simulink model "SensorModelSim"  (R2019b)
settings: Solver=VariableStepAuto  StartTime=0.0  StopTime=10.0  RelTol=1e-3
values from neighbouring files (symbols this model uses):
  A = [0  0  0  1  0  0  0  0  0  0  0  0 ... (first row only)    [LQR.m]    (also in LQR_Goal_1.m; Naman_LQR_Working.m; PlantModel.m = [0  0  0  1  0  0  0  0  0  0  0  0;      0  0  0  0  1  0  )
  B = [0      0       0       0 ... (first row only)    [LQR.m]    (also in LQR_Goal_1.m; Naman_LQR_Working.m; PlantModel.m = [0 0 0 0;      0 0 0 0;      0 0 0 0;      0 0 0 0;      0 0)
  C = [1 0 0 0 0 0 0 0 0 0 0 0 ... (first row only)    [LQR.m]    (also in LQR_Goal_1.m; Naman_LQR_Working.m; PlantModel.m = [1 0 0 0 0 0 0 0 0 0 0 0;      0 1 0 0 0 0 0 0 0 0 0 0;     )
  D = zeros(6,4)    [LQR.m]    (also in LQR_Goal_1.m; Naman_LQR_Working.m; PlantModel.m)
settings Model: Creator=Lakshu  LastModifiedBy=Sravan

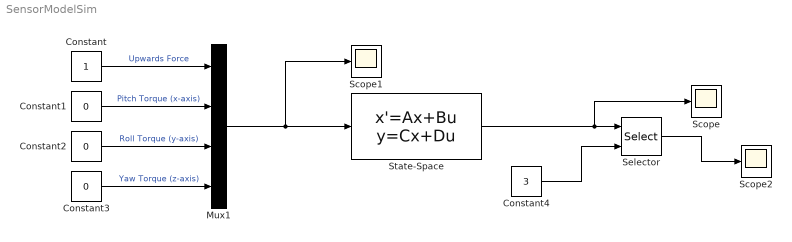
== system SensorModelSim ==
  Constant : Constant
  Constant1 : Constant  Value=0
  Constant2 : Constant  Value=0
  Constant3 : Constant  Value=0
  Constant4 : Constant  Value=3
  Mux1 : Mux
  Scope : Scope
  Scope1 : Scope
  Scope2 : Scope
  Selector : Selector  InputPortWidth=6  IndexOptions=Index vector (port)  Indices=[2]  OutputSizes=1
  State-Space : StateSpace  A=A  B=B  C=C  D=D  InitialCondition=0
  wires:
  Mux1/1 -> State-Space/1, Scope1/1
  Constant/1 -> Mux1/1  "Upwards Force"
  Constant1/1 -> Mux1/2  "Pitch Torque (x-axis)"
  Constant2/1 -> Mux1/3  "Roll Torque (y-axis)"
  Constant3/1 -> Mux1/4  "Yaw Torque (z-axis)"
  State-Space/1 -> Scope/1, Selector/1
  Constant4/1 -> Selector/2
  Selector/1 -> Scope2/1
